simulink model "AdaptiveSuspensionpid(1)"  (R2024b)
settings: Solver=ode45  StartTime=0.0  StopTime=15  MaxStep=0.001  RelTol=1e-4  AbsTol=1e-6
libraries: slpidlib x1, commrandsrc3 x1, simulink x1
settings Model: Creator=Mibra  LastModifiedBy=Mibra

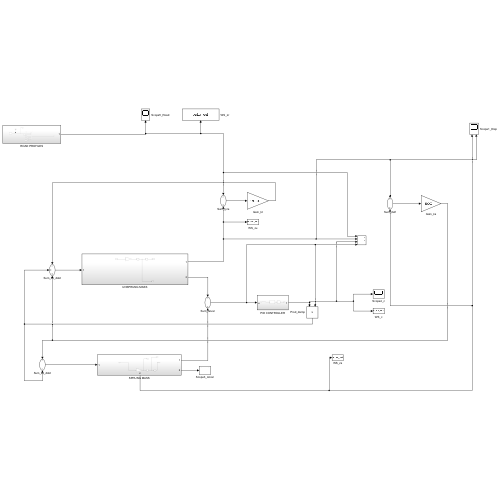
[thumbnail: Simulink's stored preview of the top-level diagram]
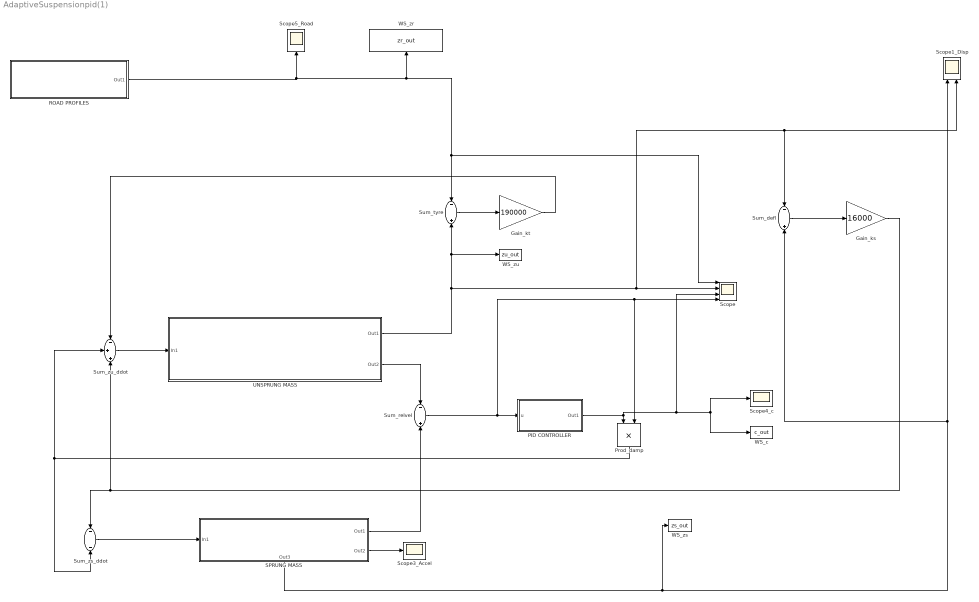
== system AdaptiveSuspensionpid(1) ==
  Gain_ks : Gain  Gain=16000
  Gain_kt : Gain  Gain=190000
  PID CONTROLLER : Subsystem
  Prod_damp : Product
  ROAD PROFILES : Subsystem
  SPRUNG MASS : Subsystem
      settings: PortSchema="{\"entries\":[{\"content\":{\"sides\":[{\"content\":{\"connectorIds\":[\"In1\"]},\"type\":\"ConnectorPlacement.EquallySpacedRectSide\",\"uuid\":\"6ad79ffb-599b-4c81-a892-dbb7801d81b8\"},{\"content\":{\"connectorIds\":[\"Out1\",\"Out2\"],\"side\":\"RIGHT\"},\"type\":\"ConnectorPlacement.EquallySpacedRectSide\",\"uuid\":\"93343421-a58f-4681-800b-8a8b239ce8f5\"},{\"content\":{\"side\":\"TOP\"},\"type\":\"ConnectorPlacement.EquallySpacedRectSide\",\"uuid\":\"5cf2d3f0-6f82-45e2-ad5d-7f515c29da59\"},{\"content\":{\"connectorIds\":[\"Out3\"],\"side\":\"BOTTOM\"},\"type\":\"ConnectorPlacement.EquallySpacedRectSide\",\"uuid\":\"0d6fe3bc-baef-47cd-bf82-e22706f5677c\"}]},\"type\":\"ConnectorPlacement.EquallySpacedConnector\",\"uuid\":\"b5841f99-fb31-46b1-8cdb-f52f1b7d9b89\"}],\"packageUris\":[\"http://schema.mathworks.com/mf0/Connector/R2020b\"],\"version\":\"1.0\"}"
  Scope : Scope  NumInputPorts=4
  Scope1_Disp : Scope  NumInputPorts=2
  Scope3_Accel : Scope
  Scope4_c : Scope
  Scope5_Road : Scope
  Sum_defl : Sum  Inputs=-+
  Sum_relvel : Sum  Inputs=-+
  Sum_tyre : Sum  Inputs=-+
  Sum_zs_ddot : Sum  Inputs=--
  Sum_zu_ddot : Sum  Inputs=-++
  UNSPRUNG MASS : Subsystem
  WS_c : ToWorkspace  VariableName=c_out  SampleTime=-1
  WS_zr : ToWorkspace  VariableName=zr_out  SampleTime=-1
  WS_zs : ToWorkspace  VariableName=zs_out  SampleTime=-1
  WS_zu : ToWorkspace  VariableName=zu_out  SampleTime=-1
  wires:
  Gain_kt/1 -> Sum_zu_ddot/1
  Gain_ks/1 -> Sum_zs_ddot/1, Sum_zu_ddot/3
  Sum_relvel/1 -> Prod_damp/2, Scope/4, PID CONTROLLER/1(u)
  Prod_damp/1 -> Sum_zu_ddot/2, Sum_zs_ddot/2
  Sum_tyre/1 -> Gain_kt/1
  Sum_defl/1 -> Gain_ks/1
  ROAD PROFILES/1(Out1) -> Scope5_Road/1, WS_zr/1, Scope/1, Sum_tyre/1
  UNSPRUNG MASS/1(Out1) -> Sum_tyre/2, WS_zu/1, Sum_defl/1, Scope1_Disp/2, Scope/2
  Sum_zu_ddot/1 -> UNSPRUNG MASS/1(In1)
  UNSPRUNG MASS/2(Out2) -> Sum_relvel/1
  SPRUNG MASS/3(Out3) -> Scope1_Disp/1, Sum_defl/2, WS_zs/1
  Sum_zs_ddot/1 -> SPRUNG MASS/1(In1)
  SPRUNG MASS/1(Out1) -> Sum_relvel/2
  SPRUNG MASS/2(Out2) -> Scope3_Accel/1
  PID CONTROLLER/1(Out1) -> Scope/3, Scope4_c/1, WS_c/1, Prod_damp/1

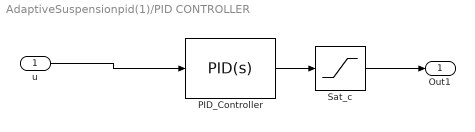
== system AdaptiveSuspensionpid(1)/PID CONTROLLER ==
  u : Inport
  PID_Controller : slpidlib/PID Controller  Controller=PID  Form=Parallel  TimeDomain=Continuous-time  UseExternalTs=off  SampleTime=-1  IntegratorMethod=Forward Euler  FilterMethod=Forward Euler  ControllerParametersSource=internal  P=2500  I=800  UseKiTs=off  D=120  UseExternalDerivativeSource=off  N=100  UseFilter=on  TunerSelectOption=Transfer Function Based (PID Tuner App)  InitialConditionSource=internal  InitialConditionForIntegrator=0  InitialConditionForFilter=0  DifferentiatorICPrevScaledInput=0  ExternalReset=none  TrackingMode=off  Kt=1  LimitOutput=off  SatLimitsSource=internal  UpperSaturationLimit=inf  LowerSaturationLimit=-inf  LinearizeAsGain=on  AntiWindupMode=clamping  Kb=1  LimitIntegrator=off  UpperIntegratorSaturationLimit=inf  LowerIntegratorSaturationLimit=-inf  POutMin=[]  POutMax=[]  IOutMin=[]  IOutMax=[]  DOutMin=[]  DOutMax=[]  NOutMin=[]  NOutMax=[]  SumOutMin=[]  SumOutMax=[]  SaturationOutMin=[]  SaturationOutMax=[]  PParamMin=[]  PParamMax=[]  IParamMin=[]  IParamMax=[]  DParamMin=[]  DParamMax=[]  NParamMin=[]  NParamMax=[]  KbParamMin=[]  KbParamMax=[]  KtParamMin=[]  KtParamMax=[]  KbOutMin=[]  KbOutMax=[]  KtOutMin=[]  KtOutMax=[]  IntegratorOutMin=[]  IntegratorOutMax=[]  FilterOutMin=[]  FilterOutMax=[]  SumI1OutMin=[]  SumI1OutMax=[]  SumI2OutMin=[]  SumI2OutMax=[]  SumI3OutMin=[]  SumI3OutMax=[]  SumI4OutMin=[]  SumI4OutMax=[]  SumDOutMin=[]  SumDOutMax=[]  DifferentiatorOutMin=[]  DifferentiatorOutMax=[]  FilterDiffOutCoefMin=[]  FilterDiffOutCoefMax=[]  ReciprocalOutMin=[]  ReciprocalOutMax=[]  SumDenOutMin=[]  SumDenOutMax=[]  SumNumOutMin=[]  SumNumOutMax=[]  DivideOutMin=[]  DivideOutMax=[]  UdiffTsProdOutMin=[]  UdiffTsProdOutMax=[]  NTsProdOutMin=[]  NTsProdOutMax=[]  UintegralTsProdOutMin=[]  UintegralTsProdOutMax=[]  UngainTsProdOutMin=[]  UngainTsProdOutMax=[]  ClampingZeroOutDataTypeStr=Inherit: Inherit via back propagation  ClampingZeroOutMin=[]  ClampingZeroOutMax=[]  FilterDenConstantOutDataTypeStr=Inherit: Inherit via back propagation  FilterDenConstantOutMin=[]  FilterDenConstantOutMax=[]  PCopyOutDataTypeStr=Inherit: Inherit via back propagation  PCopyOutMin=[]  PCopyOutMax=[]  NCopyOutDataTypeStr=Inherit: Inherit via back propagation  NCopyOutMin=[]  NCopyOutMax=[]  IntegratorContinuousStateAttributes=''  IntegratorStateMustResolveToSignalObject=off  IntegratorRTWStateStorageClass=Auto  FilterContinuousStateAttributes=''  FilterStateMustResolveToSignalObject=off  FilterRTWStateStorageClass=Auto  ParallelPVariant=InternalParameters  IdealPVariant=Disabled  IVariant=InternalParameters  DVariant=InternalParameters  IntegratorVariant=Continuous  SatVariant=Disabled  AWVariant=Passthrough  PCopyVariant=Disabled  TRVariant=Disabled  FdbkBlocksVariant=Forward  IdealPFdbkVariant=Disabled  SatFdbkVariant=Disabled  DerivativeFilterVariant=ContFilter  NVariant=InternalParameters  NCopyVariant=Disabled  FilterICVariant=InternalICsFilter  IntegratorICVariant=InternalICs  ExternalResetVariant=Disabled  TRSumVariant=Passthrough  SumFdbkVariant=Disabled  SumVariant=Sum_PID  TsampFilterVariant=InternalTs  TsampNgainVariant=Passthrough  TsampIntegralVariant=Disabled_SignalSpec  ExternalSaturationOutDataTypeStr=Inherit: Same as second input  DerivativeSourceVariant=ErrorSignal  PreIntVariant=InternalPreInt
  Sat_c : Saturate  UpperLimit=5000  LowerLimit=500
  Out1 : Outport
  wires:
  u/1 -> PID_Controller/1
  PID_Controller/1 -> Sat_c/1
  Sat_c/1 -> Out1/1

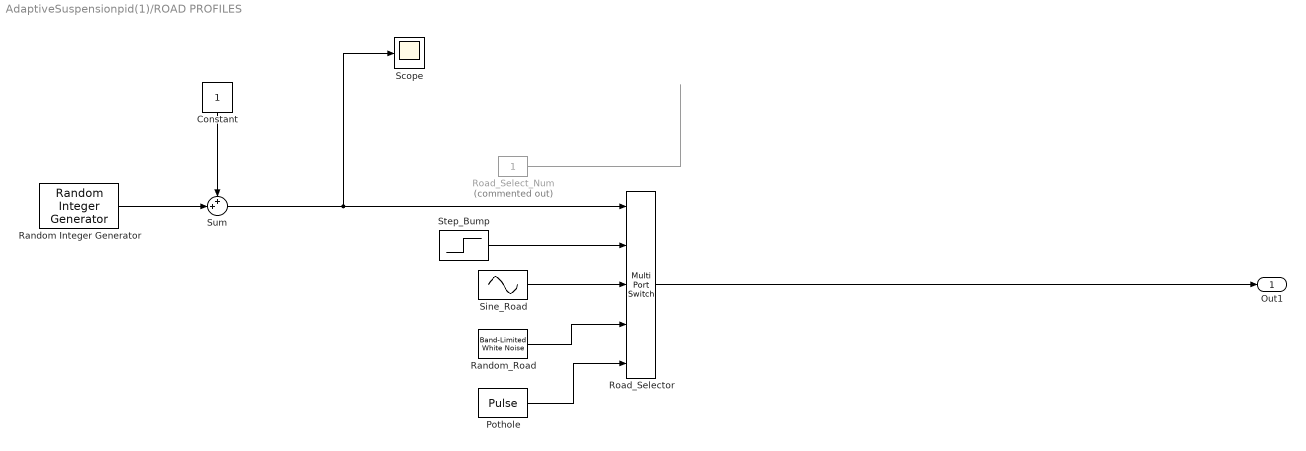
== system AdaptiveSuspensionpid(1)/ROAD PROFILES ==
  Constant : Constant
  Pothole : DiscretePulseGenerator  PulseType=Time based  Amplitude=0.08  Period=10  PulseWidth=10  PhaseDelay=2
  Random Integer Generator : commrandsrc3/Random Integer Generator  SetSize=5  SeedSource=Parameter  Seed=1  SampleTime=2  SamplesPerFrame=1  OutputDataType=single  SimulateUsing=Interpreted execution
  Random_Road : simulink/Sources/Band-Limited White Noise  Cov=0.0002  Ts=2  seed=23341
  Road_Select_Num : Constant  Commented=on
  Road_Selector : MultiPortSwitch  Inputs=4  SaturateOnIntegerOverflow=off  InputSameDT=off
  Scope : Scope
  Sine_Road : Sin  Amplitude=0.03  Frequency=12.5664  SampleTime=0
  Step_Bump : Step  After=0.05  SampleTime=0
  Sum : Sum  Inputs=++|
  Out1 : Outport
  wires:
  Sine_Road/1 -> Road_Selector/3
  Pothole/1 -> Road_Selector/5
  Random_Road/1 -> Road_Selector/4
  Step_Bump/1 -> Road_Selector/2
  Road_Select_Num/1 -> ?
  Road_Selector/1 -> Out1/1
  Constant/1 -> Sum/1
  Random Integer Generator/1 -> Sum/2
  Sum/1 -> Scope/1, Road_Selector/1

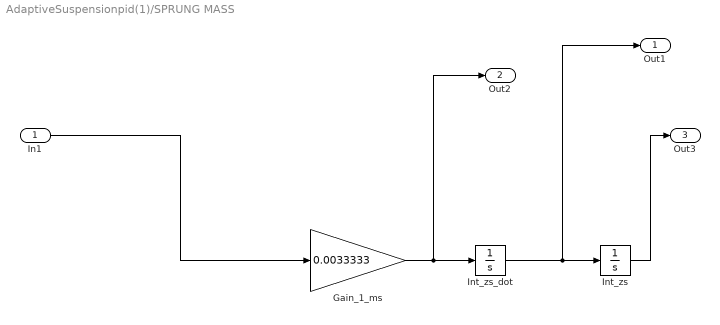
== system AdaptiveSuspensionpid(1)/SPRUNG MASS ==
  In1 : Inport
  Gain_1_ms : Gain  Gain=0.0033333
  Int_zs : Integrator
  Int_zs_dot : Integrator
  Out1 : Outport
  Out2 : Outport  Port=2
  Out3 : Outport  Port=3
  wires:
  Int_zs_dot/1 -> Out1/1, Int_zs/1
  In1/1 -> Gain_1_ms/1
  Gain_1_ms/1 -> Out2/1, Int_zs_dot/1
  Int_zs/1 -> Out3/1

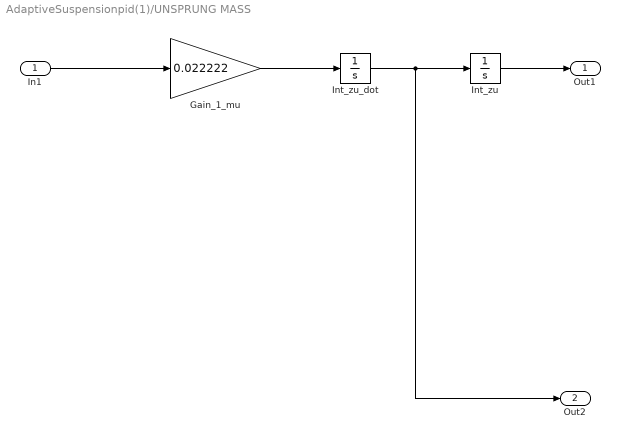
== system AdaptiveSuspensionpid(1)/UNSPRUNG MASS ==
  In1 : Inport
  Gain_1_mu : Gain  Gain=0.022222
  Int_zu : Integrator
  Int_zu_dot : Integrator
  Out1 : Outport
  Out2 : Outport  Port=2
  wires:
  In1/1 -> Gain_1_mu/1
  Int_zu_dot/1 -> Out2/1, Int_zu/1
  Gain_1_mu/1 -> Int_zu_dot/1
  Int_zu/1 -> Out1/1
